simulink model "battery_soc_estimation_ekf_ukf"  (R2023b)
settings: Solver=VariableStepAuto  StartTime=0.0  StopTime=2000  FixedStep=Ts  RelTol=1e-3  EnableMultiTasking=on
PreLoadFcn:
  | BatterySOCEstimationData;
libraries: fl_lib x4, nesl_utility x4, simulink x3, batteryecm_lib x1, BatteryEstimators x1
CloseFcn:
  | try
  |     close(h1_BatterySOCEstimation)
  | catch
  | end
  | 
  | clear h1_BatterySOCEstimation
  | 
  | clear BatterySOCEstimationSimlog
  | clear BatterySOCEstimationLogsout
  | 
  | clear AH SOC_vec T_vec R0_mat R1_mat tau1_mat
  | clear V0_mat Q R P0 initialSOC SOC0 Ts
  | clear cell_area h_conv thermal_mass
Description:
  | Battery State-of-Charge Estimation
settings Model: Creator=The MathWorks, Inc.  LastModifiedBy=muhammedalessa
settings SolverCC: AlgebraicLoopSolver=TrustRegion  AutoInsertRateTranBlk=on  MaxZcPerStep=1
settings DataIOCC: MaxDataPoints=370000  ReturnWorkspaceOutputs=off  SignalLoggingName=BatterySOCEstimationLogsout
settings OptimizationCC: ReuseModelBlockBuffer=off  LifeSpan=inf
settings DebuggingCC: UnconnectedInputMsg=warning  UnconnectedOutputMsg=warning  UnconnectedLineMsg=warning  SFUnexpectedBacktrackingDiag=warning  SFNoUnconditionalDefaultTransitionDiag=warning  SFExecutionAtInitializationDiag=none  ArithmeticOperatorsInVariantConditions=warning
settings ModelReferenceCC: EnableRefExpFcnMdlSchedulingChecks=on
settings SFSimCC: SimUseLocalCustomCode=off  CustomCodeUndefinedFunction=UseInterfaceOnly
settings RTWCC: RTWUseLocalCustomCode=off  DLArmComputeVersion=19.05
settings CodeAppCC: StateflowObjectComments=on
settings GRTTargetCC: TargetLangStandard=C89/C90 (ANSI)
settings ConfigComp: CovMetricSettings=dw  CovSaveCumulativeToWorkspaceVar=on  CovSaveSingleToWorkspaceVar=on  CovExternalEMLEnable=off
settings SimscapeCC: SimscapeLogType=all  SimscapeLogSimulationStatistics=on  SimscapeLogName=BatterySOCEstimationSimlog  SimscapeLogLimitData=off  SimscapeLogDataHistory=370000

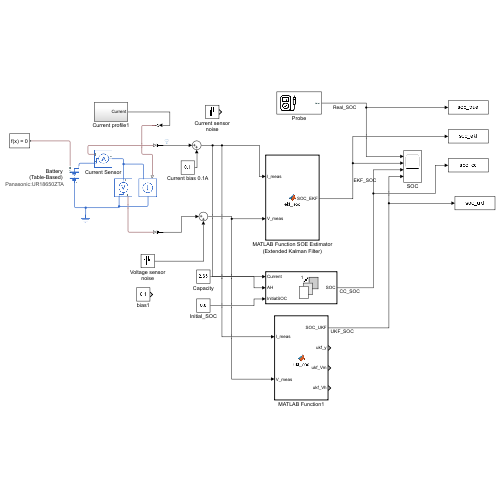
[thumbnail: Simulink's stored preview of the top-level diagram]
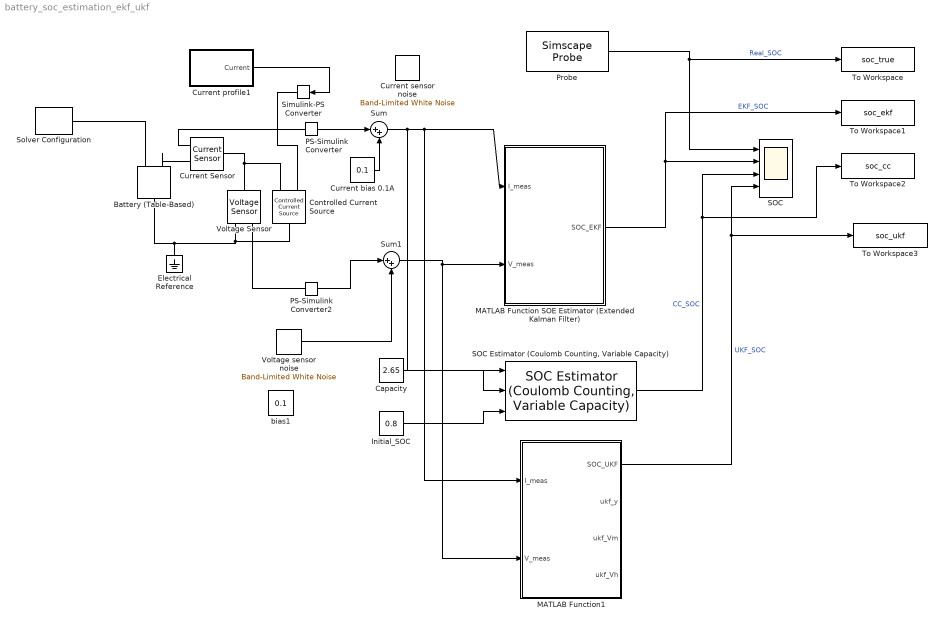
== system battery_soc_estimation_ekf_ukf ==
  Battery (Table-Based) : batteryecm_lib/Battery (Table-Based)  Tag={'toolbox/physmod/battery/shared_library/m/batteryecm_lib_parts';'Battery__Table_Based_/Panasonic/UR18650ZTA.xml'}  SOC_vec=SOC_vec  T_dependence=simscape.enum.tablebattery.temperature_dependence.yes  prm_dir=simscape.enum.tablebattery.prm_dir.noCurrentDirectionality  T_vec=[5, 20, 40] degC  V0_mat=V0_mat V  V0_vec=[3.04339 3.19969 3.32733 3.41897 3.47789 3.5189 3.54757 3.56926 3.58543 3.59715 3.60656 3.61458 3.62125 3.62859 3.63585 3.64117 3.64677 3.65281 3.65754 3.6622 3.66686 3.67118 3.67547 3.67953 3.68333 3.68679 3.68929 3.69163 3.69398 3.69633 3.69868 3.70108 3.7035 3.70592 3.70834 3.71076 3.71334 3.71599 3.71889 3.72198 3.72508 3.72817 3.73126 3.73436 3.73745 3.74054 3.74364 3.74686 3.75011 3.75346 3.75768 3.7621 3.76652 3.77094 3.77575 3.78058 3.78546 3.79147 3.79777 3.80409 3.8104 3.81672 3.82303 3.82935 3.83618 3.84344 3.8508 3.85816 3.86553 3.87289 3.88052 3.88833 3.89603 3.90423 3.91256 3.92124 3.93029 3.93933 3.94837 3.95788 3.96788 3.97854 3.98931 4.00008 4.01149 4.02304 4.03459 4.04614 4.05768 4.06947 4.08184 4.09422 4.1067 4.11982 4.1326 4.14615 4.15754 4.16699 4.17222 4.18119 4.30838] V  V_range=[2.7 Inf] V  R0_mat=R0_mat Ohm  R0_vec=[0.04577 0.0693 0.0871 0.0981 0.10274 0.10473 0.1047 0.10401 0.1029 0.10084 0.09855 0.0961 0.09374 0.0923 0.09098 0.08942 0.08829 0.08779 0.08711 0.08642 0.08573 0.08504 0.08435 0.08362 0.08285 0.0821 0.08136 0.08067 0.07998 0.07929 0.07859 0.07791 0.07723 0.07655 0.07588 0.0752 0.07463 0.07414 0.07372 0.07333 0.07295 0.07256 0.07218 0.07179 0.07141 0.07102 0.07064 0.07034 0.07007 0.06981 0.06973 0.0697 0.06966 0.06963 0.06966 0.06969 0.06974 0.07 0.07016 0.07032 0.07047 0.07062 0.07078 0.07093 0.07117 0.0715 0.07186 0.07221 0.07256 0.07292 0.07332 0.07375 0.0741 0.07448 0.07489 0.07535 0.07584 0.07633 0.07682 0.07759 0.07866 0.07988 0.08112 0.08236 0.08368 0.08499 0.0863 0.08761 0.08891 0.09039 0.09225 0.09411 0.09597 0.09796 0.0995 0.10104 0.10043 0.09826 0.09216 0.08512 0.00997] Ohm  R0_dis_mat=[.0117, .0085, .009; .011, .0085, .009; .0114, .0087, .0092; .0107, .0082, .0088; .0107, .0083, .0091; .0113, .0085, .0089; .0116, .0085, .0089] % Parameter not set Ohm  R0_dis_vec=[.0085, .0085, .0087, .0082, .0083, .0085, .0085] % Parameter not set Ohm  R0_ch_mat=[.0117, .0085, .009; .011, .0085, .009; .0114, .0087, .0092; .0107, .0082, .0088; .0107, .0083, .0091; .0113, .0085, .0089; .0116, .0085, .0089] % Parameter not set Ohm  R0_ch_vec=[.0085, .0085, .0087, .0082, .0083, .0085, .0085] % Parameter not set Ohm  AH=2.65 hr*A  prm_leak=simscape.enum.tablebattery.prm_leak.disabled  Rleak_vec=[8000, 7000, 6000] % Parameter not set Ohm  Rleak=7e3 % Parameter not set Ohm  extrapolation_option=simscape.enum.extrapolation.nearest  SOC_port=simscape.enum.tablebattery.enable.yes  prm_dyn=simscape.enum.tablebattery.prm_dyn.rc1  R1_mat=R1_mat Ohm  R1_vec=[.0029, .0024, .0026, .0016, .0023, .0018, .0017] % Parameter not set Ohm  tau1_mat=tau1_mat s  tau1_vec=[36, 45, 105, 29, 77, 33, 39] % Parameter not set s  R2_mat=[.0109, .0029, .0013; .0069, .0024, .0012; .0047, .0026, .0013; .0034, .0016, .001; .0033, .0023, .0014; .0033, .0018, .0011; .0028, .0017, .0011] % Parameter not set Ohm  R2_vec=[.0029, .0024, .0026, .0016, .0023, .0018, .0017] % Parameter not set Ohm  tau2_mat=[20, 36, 39; 31, 45, 39; 109, 105, 61; 36, 29, 26; 59, 77, 67; 40, 33, 29; 25, 39, 33] % Parameter not set s  tau2_vec=[36, 45, 105, 29, 77, 33, 39] % Parameter not set s  R3_mat=[.0109, .0029, .0013; .0069, .0024, .0012; .0047, .0026, .0013; .0034, .0016, .001; .0033, .0023, .0014; .0033, .0018, .0011; .0028, .0017, .0011] % Parameter not set Ohm  R3_vec=[.0029, .0024, .0026, .0016, .0023, .0018, .0017] % Parameter not set Ohm  tau3_mat=[20, 36, 39; 31, 45, 39; 109, 105, 61; 36, 29, 26; 59, 77, 67; 40, 33, 29; 25, 39, 33] % Parameter not set s  tau3_vec=[36, 45, 105, 29, 77, 33, 39] % Parameter not set s  R4_mat=[.0109, .0029, .0013; .0069, .0024, .0012; .0047, .0026, .0013; .0034, .0016, .001; .0033, .0023, .0014; .0033, .0018, .0011; .0028, .0017, .0011] % Parameter not set Ohm  R4_vec=[.0029, .0024, .0026, .0016, .0023, .0018, .0017] % Parameter not set Ohm  tau4_mat=[20, 36, 39; 31, 45, 39; 109, 105, 61; 36, 29, 26; 59, 77, 67; 40, 33, 29; 25, 39, 33] % Parameter not set s  tau4_vec=[36, 45, 105, 29, 77, 33, 39] % Parameter not set s  R5_mat=[.0109, .0029, .0013; .0069, .0024, .0012; .0047, .0026, .0013; .0034, .0016, .001; .0033, .0023, .0014; .0033, .0018, .0011; .0028, .0017, .0011] % Parameter not set Ohm  R5_vec=[.0029, .0024, .0026, .0016, .0023, .0018, .0017] % Parameter not set Ohm  tau5_mat=[20, 36, 39; 31, 45, 39; 109, 105, 61; 36, 29, 26; 59, 77, 67; 40, 33, 29; 25, 39, 33] % Parameter not set s  tau5_vec=[36, 45, 105, 29, 77, 33, 39] % Parameter not set s  prm_fade=simscape.enum.tablebattery.prm_fade.tableN  N0=100 % Parameter not set  dV0=0 % Parameter not set  dR0=0 % Parameter not set  dAH=0 % Parameter not set  dRleak=0 % Parameter not set  dR1=0 % Parameter not set  dR2=0 % Parameter not set  dR3=0 % Parameter not set  dR4=0 % Parameter not set  dR5=0 % Parameter not set  N0vec=[0 7 13 19 25 31 37 43 49 55 61 67 73 79 85 91 97 103 109 115 121 127 133 139 145 151 157 163 169 175 181 187 193 199 205 211 217 223 229 235 241 247 253 259 265 271 277 283 289 295 301 307 313 319 325 331 337 343 349 355 361 367 373 379 385 391 397 403 409 415 421 427 433 439 445 451 457 463 469 475 481 487 493 499]  Tfadevec=[298.15, 323.15] % Parameter not set K  dV0vec=[0 -1.7373 -2.9889 -3.1115 -3.2033 -3.2746 -3.3973 -3.5142 -3.6524 -3.7953 -3.9595 -4.1213 -4.2764 -4.433 -4.5902 -4.7179 -4.8412 -4.9645 -5.0868 -5.209 -5.3312 -5.4534 -5.5742 -5.6906 -5.807 -5.9213 -6.0353 -6.1494 -6.2635 -6.3776 -6.4816 -6.5242 -6.5668 -6.6094 -6.6519 -6.6945 -6.7371 -6.7797 -6.8223 -6.8649 -6.9072 -6.9493 -6.9914 -7.0334 -7.0755 -7.1175 -7.1552 -7.187 -7.2188 -7.2507 -7.2825 -7.3143 -7.3461 -7.3779 -7.4097 -7.4415 -7.4714 -7.4908 -7.5103 -7.5297 -7.5491 -7.5685 -7.588 -7.6074 -7.6268 -7.6463 -7.6656 -7.6848 -7.7105 -7.7394 -7.7683 -7.7971 -7.826 -7.8549 -7.8838 -7.9121 -7.9392 -7.9554 -7.9697 -7.9841 -7.9984 -8.0127 -8.0271 -8.0414]  dR0vec=zeros(1, 84)  dAHvec=[0 -0.588 -1.177 -1.765 -2.354 -2.942 -3.527 -4.05 -4.572 -5.095 -5.617 -6.14 -6.662 -7.185 -7.701 -8.127 -8.553 -8.978 -9.404 -9.829 -10.255 -10.68 -11.106 -11.532 -11.957 -12.383 -12.808 -13.234 -13.659 -14.085 -14.473 -14.632 -14.791 -14.95 -15.109 -15.267 -15.426 -15.585 -15.744 -15.903 -16.062 -16.221 -16.379 -16.538 -16.697 -16.856 -16.998 -17.125 -17.253 -17.38 -17.507 -17.634 -17.762 -17.889 -18.016 -18.143 -18.263 -18.341 -18.418 -18.496 -18.574 -18.651 -18.729 -18.807 -18.885 -18.962 -19.04 -19.118 -19.221 -19.338 -19.455 -19.572 -19.688 -19.805 -19.922 -20.039 -20.156 -20.225 -20.287 -20.349 -20.41 -20.472 -20.534 -20.596]  dRleakvec=[0, 0, 0] % Parameter not set  dR1vec=zeros(1, 84)  dR2vec=[0, 0, 0] % Parameter not set  dR3vec=[0, 0, 0] % Parameter not set  dR4vec=[0, 0, 0] % Parameter not set  dR5vec=[0, 0, 0] % Parameter not set  dV0mat=[0, 0; 0, 0; 0, 0] % Parameter not set  dR0mat=[0, 0; 0, 0; 0, 0] % Parameter not set  dAHmat=[0, 0; 0, 0; 0, 0] % Parameter not set  dRleakmat=[0, 0; 0, 0; 0, 0] % Parameter not set  dR1mat=[0, 0; 0, 0; 0, 0] % Parameter not set  dR2mat=[0, 0; 0, 0; 0, 0] % Parameter not set  dR3mat=[0, 0; 0, 0; 0, 0] % Parameter not set  dR4mat=[0, 0; 0, 0; 0, 0] % Parameter not set  dR5mat=[0, 0; 0, 0; 0, 0] % Parameter not set  prm_age_modeling=simscape.enum.tablebattery.prm_age_modeling.equation  storage_dt_age_vec=[0] % Parameter not set d  storage_T_age_vec=[273] % Parameter not set K  prm_age_OCV=simscape.enum.tablebattery.prm_age_OCV.OCV  OCV_age=0.9 % Parameter not set  SOC_age=0.6 % Parameter not set  prm_age_resistance=simscape.enum.tablebattery.prm_age.disabled  OCV_scaling_age_resistance=2.2134e6 % Parameter not set  OCV_offset_age_resistance=1.632e6 % Parameter not set  temp_exp_age_resistance=0.515833569 % Parameter not set V  t_exp_age_resistance=0.75 % Parameter not set  T_age_vec_resistance=[273.15, 298.15, 323.15] % Parameter not set K  dt_age_vec_resistance=[90, 180, 270, 360] % Parameter not set d  dR0_age_vec=[0, 0, 0] % Parameter not set  t_meas_dR0_age=100 % Parameter not set d  dR0_age_mat=[0, 0, 0; 0, 0, 0; 0, 0, 0; 0, 0, 0] % Parameter not set  prm_age_capacity=simscape.enum.tablebattery.prm_age.disabled  OCV_scaling_age_capacity=1.5097e07 % Parameter not set  OCV_offset_age_capacity=8.3625e06 % Parameter not set  temp_exp_age_capacity=0.6011 % Parameter not set V  t_exp_age_capacity=0.75 % Parameter not set  T_age_vec_capacity=[273.15, 298.15, 323.15] % Parameter not set K  dt_age_vec_capacity=[90, 180, 270, 360] % Parameter not set d  dAH_age_vec=[0, 0, 0] % Parameter not set  t_meas_dAH_age=100 % Parameter not set d  dAH_age_mat=[0, 0, 0; 0, 0, 0; 0, 0, 0; 0, 0, 0] % Parameter not set  thermal_port=simscape.enum.thermaleffects.omit  temperature=298.15 % Parameter not set K  thermal_mass=44.1 % Parameter assumed J/K  i_specify=off  i_priority=None  i=0 A  i_nominal_specify=off  i_nominal_unit=A  i_nominal_value=1  v_specify=off  v_priority=None  v=0 V  v_nominal_specify=off  v_nominal_unit=V  v_nominal_value=1  stateOfCharge_specify=off  stateOfCharge_priority=High  stateOfCharge=initialSOC  stateOfCharge_nominal_specify=off  stateOfCharge_nominal_unit=1  stateOfCharge_nominal_value=1  num_cycles_specify=off  num_cycles_priority=High  num_cycles=0  num_cycles_nominal_specify=off  num_cycles_nominal_unit=1  num_cycles_nominal_value=1  cell_temperature_specify=off  cell_temperature_priority=High  cell_temperature=293.15 K  cell_temperature_nominal_specify=off  cell_temperature_nominal_unit=K  cell_temperature_nominal_value=1
      settings: AttributesFormatString=Panasonic:UR18650ZTA  InternalSimscapePortConfiguration="{\"Bottom\":[],\"Left\":[{\"id\":\"p\",\"label\":\"+\",\"type\":\"foundation.electrical.electrical\"},{\"id\":\"soc\",\"label\":\"SOC\",\"type\":\"output\"}],\"Right\":[{\"id\":\"n\",\"label\":\"-\",\"type\":\"foundation.electrical.electrical\"}],\"Top\":[]}"
  Capacity : Constant  Value=2.65
  Controlled Current Source : fl_lib/Electrical/Electrical Sources/Controlled Current Source
  Current Sensor : fl_lib/Electrical/Electrical Sensors/Current Sensor
  Current bias 0.1A : Constant  Value=0.1
  Current profile1 : Subsystem
  Current sensor noise : simulink/Sources/Band-Limited White Noise  Cov=1e-2  Ts=1  seed=1234
  Electrical Reference : fl_lib/Electrical/Electrical Elements/Electrical Reference
  Initial_SOC : Constant  Value=0.8
  MATLAB Function SOE Estimator (Extended Kalman Filter) : MATLAB Function  TreatAsAtomicUnit=on
  MATLAB Function1 : MATLAB Function  TreatAsAtomicUnit=on
  PS-Simulink Converter : nesl_utility/PS-Simulink Converter  PhysicalDomain=network_engine_domain  SubClassName=ps_output  LeftPortType=input  RightPortType=output  PseudoPeriodic=off  Frequencies=[]  VectorFormat=inherit  Unit=inherit  AffineConversion=off
  PS-Simulink Converter2 : nesl_utility/PS-Simulink Converter  PhysicalDomain=network_engine_domain  SubClassName=ps_output  LeftPortType=input  RightPortType=output  PseudoPeriodic=off  Frequencies=[]  VectorFormat=inherit  Unit=inherit  AffineConversion=off
  Probe : SimscapeProbe  BoundBlock=1225  Variables={soc}
  SOC : Scope  NumInputPorts=4
  "SOC Estimator (Coulomb Counting, Variable Capacity)" : BatteryEstimators/SOC Estimator (Coulomb Counting, Variable Capacity)  CurrentInputPartition=off  Ts=1
      settings: LibrarySourceBlock=|
      | batt_sl_lib/Estimators/SOC Estimator
      | (Coulomb Counting, Variable Capacity)
  Simulink-PS Converter : nesl_utility/Simulink-PS Converter  PhysicalDomain=network_engine_domain  SubClassName=ps_input  LeftPortType=input  RightPortType=output  PseudoPeriodic=off  Frequencies=[]  NoiseDistribution=none  NoiseParameters=[]  Unit=1  AffineConversion=off  FilteringAndDerivatives=provide  SimscapeFilterOrder=1  InputFilterTimeConstant=0.001  UdotUserProvided=0
  Solver Configuration : nesl_utility/Solver Configuration  PhysicalDomain=network_engine_domain  SubClassName=solver  LeftPortType=input  RightPortType=generic  Tones=[]  Harmonics=[]  SimulateNoise=off  Profile=off  UseLocalSampling=off  EnableSwitchedLinearOptims=on  FrequencyDomain=off  UseCCode=off  RelTol=0.001  AbsTol=0.001  MinStep=1e-09  ToWorkspace=off  RevertToSquareIcSolve=off  NumHomotopyIterations=100  PhasorMode=off  PhasorModeNumHarmonics=1  ConsistencySolver=NEWTON_XTOL_AFTER_FTOL  IndexReductionMethod=DerivativeReplacement  DoDC=off  ResidualTolerance=1e-09  ConsistencyTolSource=GLOBAL  ConsistencyAbsTol=0.001  ConsistencyRelTol=0.001  ConsistencyTolFactor=0.001  UseLocalSolver=off  LocalSolverChoice=NE_BACKWARD_EULER_ADVANCER  ResolveIndetEquations=on  FunctionEvalNumThread=1  LocalSolverSampleTime=0.001  DoFixedCost=off  MaxNonlinIter=3  MaxModeIter=2  ComputeImpulses=off  ImpulseIterations=2  LinearAlgebra=auto  LinearAlgebraNumThread=0  EquationFormulation=NE_TIME_EF  DelaysMemoryBudget=1024  AutomaticFiltering=on  FilteringTimeConstant=0.001  PartitionStorageMethod=AS_NEEDED  PartitionMemoryBudget=1024  PartitionMethod=ROBUST  MultibodyUseLocalSolver=off  MultibodyLocalSolverChoice=ODE1  MultibodyLocalSolverSampleTime=0.001
  Sum : Sum  Inputs=|++
  Sum1 : Sum  Inputs=|++
  To Workspace : ToWorkspace  VariableName=soc_true  SaveFormat=Timeseries  SampleTime=-1
  To Workspace1 : ToWorkspace  VariableName=soc_ekf  SaveFormat=Timeseries  SampleTime=-1
  To Workspace2 : ToWorkspace  VariableName=soc_cc  SaveFormat=Timeseries  SampleTime=-1
  To Workspace3 : ToWorkspace  VariableName=soc_ukf  SaveFormat=Timeseries  SampleTime=-1
  Voltage Sensor : fl_lib/Electrical/Electrical Sensors/Voltage Sensor
  Voltage sensor noise : simulink/Sources/Band-Limited White Noise  Cov=1e-2  Ts=1  seed=1234
  bias1 : Constant  Value=0.1
  wires:
  MATLAB Function SOE Estimator (Extended Kalman Filter)/1(SOC_EKF) -> To Workspace1/1, SOC/2  "EKF_SOC"
  Current profile1/1(Current) -> Simulink-PS Converter/1
  Probe/1 -> SOC/1, To Workspace/1  "Real_SOC"
  Capacity/1 -> "SOC Estimator (Coulomb Counting, Variable Capacity)"/2
  Initial_SOC/1 -> "SOC Estimator (Coulomb Counting, Variable Capacity)"/3
  "SOC Estimator (Coulomb Counting, Variable Capacity)"/1 -> To Workspace2/1, SOC/3  "CC_SOC"
  PS-Simulink Converter2/1 -> Sum1/1
  Sum1/1 -> MATLAB Function1/2(V_meas), MATLAB Function SOE Estimator (Extended Kalman Filter)/2(V_meas)
  Sum/1 -> MATLAB Function1/1(I_meas), MATLAB Function SOE Estimator (Extended Kalman Filter)/1(I_meas), "SOC Estimator (Coulomb Counting, Variable Capacity)"/1
  PS-Simulink Converter/1 -> Sum/1
  MATLAB Function1/1(SOC_UKF) -> To Workspace3/1, SOC/4  "UKF_SOC"
  Current bias 0.1A/1 -> Sum/2
  Voltage sensor noise/1 -> Sum1/2
  connections:
  Electrical Reference/LConn1 -- Controlled Current Source/LConn1 -- Voltage Sensor/RConn2 -- Battery (Table-Based)/RConn1
  Current Sensor/LConn1 -- Controlled Current Source/RConn2 -- Voltage Sensor/LConn1
  Voltage Sensor/RConn1 -- PS-Simulink Converter2/LConn1
  Battery (Table-Based)/LConn1 -- Current Sensor/RConn2
  PS-Simulink Converter/LConn1 -- Current Sensor/RConn1
  Controlled Current Source/RConn1 -- Simulink-PS Converter/RConn1
  Battery (Table-Based)/LConn2 -- Solver Configuration/RConn1

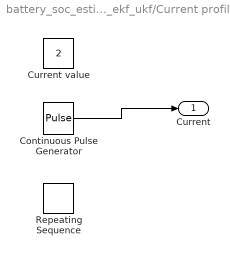
== system battery_soc_estimation_ekf_ukf/Current profile1 ==
  Continuous Pulse Generator : DiscretePulseGenerator  PulseType=Time based  Amplitude=3  Period=30  PulseWidth=33
  Current value : Constant  Value=2
  Repeating Sequence : simulink/Sources/Repeating Sequence  rep_seq_t=[0 20 30 50 60]  rep_seq_y=[0 0 3 3 0]
  Current : Outport
  wires:
  Continuous Pulse Generator/1 -> Current/1

== matlab function battery_soc_estimation_ekf_ukf/MATLAB Function1 ==
  settings: updateMethod=DISCRETE
  data: I_meas input; SOC_UKF output; V_meas input; ukf_y output; ukf_Vm output; ukf_Vh output
function [SOC_UKF, ukf_y, ukf_Vm, ukf_Vh] = ukf_soc(I_meas, V_meas)
%#codegen
% ---- Parameters (Panasonic UR18650ZTA) ----
Q_nom  = 2.65 * 3600;
dt     = 1;

SOC_bp = [0, 0.1, 0.25, 0.5, 0.75, 0.9, 1];
OCV_bp = [3.50, 3.57, 3.63, 3.71, 3.93, 4.08, 4.19];
R0_bp  = [0.0085, 0.0085, 0.0087, 0.0082, 0.0083, 0.0085, 0.0085];
R1_bp  = [0.0029, 0.0024, 0.0026, 0.0016, 0.0023, 0.0018, 0.0017];
tau_bp = [36, 45, 29, 77, 33, 33, 39];

% ---- Persistent state ----
persistent x P initialized
if isempty(initialized)
    SOC_init = 0.8;           % Same starting point as EKF for fair comparison
    x = [SOC_init; 0];
    P = diag([0.1, 1e-4]);
    initialized = true;
end

% ---- Tuning (same as EKF) ----
Q_cov = diag([1e-5, 1e-5]);
R_cov = 0.01;

% ---- UKF sigma-point parameters ----
n = 2;                    % state dimension
alpha = 1e-3;
beta  = 2;
kappa = 0;
lambda = alpha^2 * (n + kappa) - n;

% Weights for mean and covariance
Wm = zeros(1, 2*n + 1);
Wc = zeros(1, 2*n + 1);
Wm(1) = lambda / (n + lambda);
Wc(1) = Wm(1) + (1 - alpha^2 + beta);
for i = 2:(2*n + 1)
    Wm(i) = 1 / (2 * (n + lambda));
    Wc(i) = Wm(i);
end

% ---- Generate sigma points ----
% Use Cholesky; add tiny jitter for numerical stability
% Ensure P is symmetric and positive definite
P_safe = (P + P') / 2 + 1e-8 * eye(n);
L = chol((n + lambda) * P_safe, 'lower');

X = zeros(n, 2*n + 1);
X(:, 1) = x;
for i = 1:n
    X(:, i + 1)     = x + L(:, i);
    X(:, i + n + 1) = x - L(:, i);
end

% ---- Propagate sigma points through state equations ----
X_pred = zeros(n, 2*n + 1);
for i = 1:(2*n + 1)
    soc_i = min(max(X(1, i), 0.001), 0.999);
    R1_i   = interp1(SOC_bp, R1_bp, soc_i, 'linear', 'extrap');
    tau_i  = interp1(SOC_bp, tau_bp, soc_i, 'linear', 'extrap');
    a_i    = exp(-dt / tau_i);
    b_i    = R1_i * (1 - a_i);
    
    X_pred(1, i) = X(1, i) + (dt / Q_nom) * I_meas;
    X_pred(2, i) = a_i * X(2, i) - b_i * I_meas;
end

% ---- Predicted mean and covariance ----
x_pred = X_pred * Wm';
P_pred = Q_cov;
for i = 1:(2*n + 1)
    diff_x = X_pred(:, i) - x_pred;
    P_pred = P_pred + Wc(i) * (diff_x * diff_x');
end

% ---- Propagate sigma points through measurement equation ----
Y_pred = zeros(1, 2*n + 1);
for i = 1:(2*n + 1)
    soc_i = min(max(X_pred(1, i), 0.001), 0.999);
    R0_i  = interp1(SOC_bp, R0_bp, soc_i, 'linear', 'extrap');
    OCV_i = interp1(SOC_bp, OCV_bp, soc_i, 'linear', 'extrap');
    Y_pred(i) = OCV_i + R0_i * I_meas - X_pred(2, i);
end

% ---- Predicted measurement mean and covariances ----
y_pred = Y_pred * Wm';

S = R_cov;
Pxy = zeros(n, 1);
for i = 1:(2*n + 1)
    diff_y = Y_pred(i) - y_pred;
    diff_x = X_pred(:, i) - x_pred;
    S   = S + Wc(i) * (diff_y * diff_y);
    Pxy = Pxy + Wc(i) * (diff_x * diff_y);
end

% ---- Kalman gain and update ----
K = Pxy / S;
innovation = V_meas - y_pred;
x = x_pred + K * innovation;
P = P_pred - K * S * K';

% Clamp SOC
x(1) = min(max(x(1), 0), 1);

% ---- Outputs ----
SOC_UKF = x(1);
ukf_y   = innovation;
ukf_Vm  = V_meas;
ukf_Vh  = y_pred;
end

== matlab function battery_soc_estimation_ekf_ukf/MATLAB Function SOE Estimator (Extended Kalman Filter) ==
  settings: updateMethod=DISCRETE
  data: I_meas input; SOC_EKF output; V_meas input
function SOC_EKF  = ekf_soc(I_meas, V_meas)
%#codegen
Q_nom  = 2.65 * 3600;
dt     = 1;
SOC_bp = [0, 0.1, 0.25, 0.5, 0.75, 0.9, 1];
OCV_bp = [3.50, 3.57, 3.63, 3.71, 3.93, 4.08, 4.19];
R0_bp  = [0.0085, 0.0085, 0.0087, 0.0082, 0.0083, 0.0085, 0.0085];
R1_bp  = [0.0029, 0.0024, 0.0026, 0.0016, 0.0023, 0.0018, 0.0017];
tau_bp = [36, 45, 29, 77, 33, 33, 39];

persistent x P initialized
if isempty(initialized)
    SOC_init = 0.8;    % was 0.5 — EKF starts WRONG (30% too high)
    x = [SOC_init; 0];
    P = diag([0.1, 1e-4]);
    initialized = true;
end

soc_c = min(max(x(1), 0.001), 0.999);
R0   = interp1(SOC_bp, R0_bp, soc_c, 'linear', 'extrap');
R1   = interp1(SOC_bp, R1_bp, soc_c, 'linear', 'extrap');
tau1 = interp1(SOC_bp, tau_bp, soc_c, 'linear', 'extrap');
OCV  = interp1(SOC_bp, OCV_bp, soc_c, 'linear', 'extrap');

ds = 0.005;
s_hi = min(soc_c + ds, 1);
s_lo = max(soc_c - ds, 0);
dOCV = (interp1(SOC_bp, OCV_bp, s_hi, 'linear', 'extrap') - ...
        interp1(SOC_bp, OCV_bp, s_lo, 'linear', 'extrap')) / (s_hi - s_lo);

Q_cov = diag([1e-5, 1e-5]);
R_cov = 0.01;

a = exp(-dt / tau1);
b = R1 * (1 - a);
SOC_pred = x(1) + (dt / Q_nom) * I_meas;
VRC_pred = a * x(2) - b * I_meas;
x_pred = [SOC_pred; VRC_pred];

F = [1, 0; 0, a];
P_pred = F * P * F' + Q_cov;

V_hat = OCV + R0 * I_meas - VRC_pred;
y = V_meas - V_hat;
H = [dOCV, -1];
S = H * P_pred * H' + R_cov;
K = (P_pred * H') / S;

x = x_pred + K * y;
P = (eye(2) - K * H) * P_pred;
x(1) = min(max(x(1), 0), 1);

SOC_EKF = x(1);
debug_y = y;
debug_Vm = V_meas;
debug_Vh = V_hat;
end
